simulink model "Temporal4"  (R2020a)
settings: Solver=VariableStepAuto  StartTime=0.0  StopTime=1.0  RelTol=1e-3
settings Model: Creator=86188  LastModifiedBy=bzhan
settings DataIOCC: ReturnWorkspaceOutputs=off
settings DebuggingCC: ArithmeticOperatorsInVariantConditions=warning
settings SFSimCC: SimUseLocalCustomCode=off  CustomCodeUndefinedFunction=UseInterfaceOnly
settings RTWCC: RTWUseLocalCustomCode=off

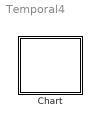
== system Temporal4 ==
  Chart : Stateflow chart  TreatAsAtomicUnit=on

== stateflow chart Temporal4/Chart ==
  settings: updateMethod=DISCRETE  sampleTime=0.1
  state A
    en:f("en_A");
    x=1;
    du:f("du_A");
    x=x+1;
  state B
    en:f("en_B")
    x=1;
    du:f("du_B");
    x=x+1;
  (default) -> A
  A -> B : before(4,tick)[x>=3]
  B -> A : before(4,tick)[x>=4]
  data: s function_input; x local
  function f(s):
    | function f(s)
    |   fprintf(s+"\n");
